simulink model "test"  (R2024b)
settings: Solver=VariableStepAuto  StartTime=0.0  StopTime=10.0  RelTol=1e-3
libraries: spsSeriesRLCLoadLib x6, spsAsynchronousMachineSIUnitsLib x4, spsUniversalBridgeLib x3, spsCurrentMeasurementLib x1, spsThreePhaseVIMeasurementLib x1, spsVoltageMeasurementLib x1
settings Model: Creator=HFUT2  LastModifiedBy=HFUT2

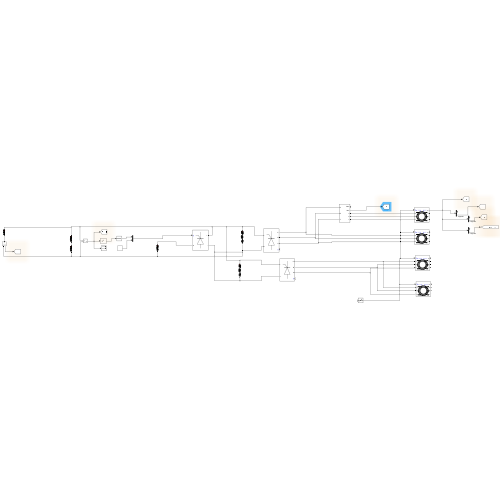
[thumbnail: Simulink's stored preview of the top-level diagram]
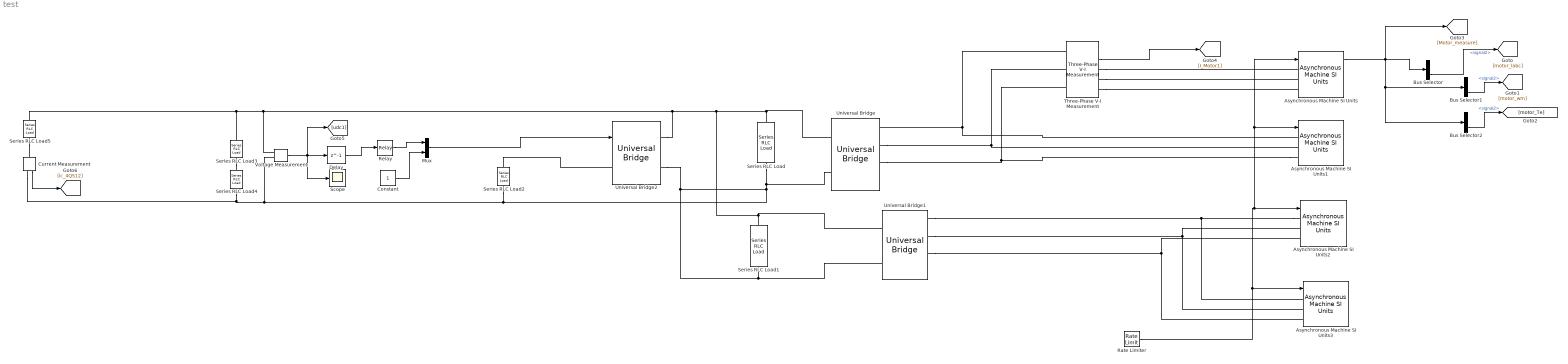
== system test ==
  Asynchronous Machine SI Units{,1..3} (4 alike) : spsAsynchronousMachineSIUnitsLib/Asynchronous Machine SI Units  RotorType=Wound  PresetModel=No  MechanicalLoad=Torque Tm  ShowDetailedParameters=on  ReferenceFrame=Rotor  Units=SI  MeasurementBus=off  NominalParameters=[1.845e+04 400 50]  VoltageRatio=1  Stator=[0.5968 0.0003495]  Rotor=[0.6258 0.005473]  Cage1=[0.4155 0.002066]  Cage2=[0.4168 0.0003495]  Lm=0.0354  Mechanical=[0.05 0.005879 2]  PolePairs=2  InitialConditions=[0 0 0 0 0 0 0 0]  SimulateSaturation=off  Saturation=[14.03593122, 27.81365428, 53.79336849, 72.68890987, 97.98006896, 148.6815601, 215.7428561, 302.9841135, 428.7778367 ; 230, 322, 414, 460, 506, 552, 598, 644, 690]  LoadFlowParameters=1492000  TsPowergui=0  TsBlock=-1  IterativeModel=Trapezoidal non iterative  IterativeDiscreteModel=Trapezoidal non iterative  Pmec=1.492e+006
  Bus Selector : BusSelector  OutputSignals=signal1,signal2
  Bus Selector1 : BusSelector  OutputSignals=signal1,signal2
  Bus Selector2 : BusSelector  OutputSignals=signal1,signal2
  Constant : Constant
  Current Measurement : spsCurrentMeasurementLib/Current Measurement  PhasorSimulation=off  OutputType=Complex  PSBequivalent=0
  Delay : Delay  DelayLength=1  InitialCondition=0
  Mux : Mux  Inputs=2
  Rate Limiter : RateLimiter  SampleTimeMode=inherited
  Relay : Relay
  Scope : Scope
  Series RLC Load{,1..5} (6 alike) : spsSeriesRLCLoadLib/Series RLC Load  LConnTagsString=a  RConnTagsString=__new0  NominalVoltage=1000  NominalFrequency=60  ActivePower=10e3  InductivePower=100  CapacitivePower=100  Setx0=off  InitialVoltage=0  SetiL0=off  InitialCurrent=0  Measurements=None  LoadType=constant Z
  Three-Phase V-I Measurement : spsThreePhaseVIMeasurementLib/Three-Phase V-I Measurement  VoltageMeasurement=phase-to-ground  SetLabelV=off  LabelV=Vabc  Vpu=off  VpuLL=off  CurrentMeasurement=yes  SetLabelI=off  LabelI=Iabc  Ipu=off  Pbase=100e6  Vbase=500e3  OutputType=Complex  PhasorSimulation=off  PSBequivalent=0
  Universal Bridge : spsUniversalBridgeLib/Universal Bridge  Arms=3  SnubberResistance=1e5  SnubberCapacitance=inf  Device=Thyristors  Ron=1e-3  Lon=0  ForwardVoltages="[  0  0  ]"  ForwardVoltage=0  GTOparameters=[ 10e-6 , 20e-6 ]  IGBTparameters=[ 1e-6 , 2e-6 ]  Measurements=None  Measurements_2=None  converterType=Rectifier
  Universal Bridge1 : spsUniversalBridgeLib/Universal Bridge  Arms=3  SnubberResistance=1e5  SnubberCapacitance=inf  Device=Thyristors  Ron=1e-3  Lon=0  ForwardVoltages="[  0  0  ]"  ForwardVoltage=0  GTOparameters=[ 10e-6 , 20e-6 ]  IGBTparameters=[ 1e-6 , 2e-6 ]  Measurements=None  Measurements_2=None  converterType=Rectifier
  Universal Bridge2 : spsUniversalBridgeLib/Universal Bridge  Arms=1  SnubberResistance=1e5  SnubberCapacitance=inf  Device=Thyristors  Ron=1e-3  Lon=0  ForwardVoltages="[  0  0  ]"  ForwardVoltage=0  GTOparameters=[ 10e-6 , 20e-6 ]  IGBTparameters=[ 1e-6 , 2e-6 ]  Measurements=None  Measurements_2=None  converterType=Rectifier
  Voltage Measurement : spsVoltageMeasurementLib/Voltage Measurement  PhasorSimulation=off  OutputType=Complex  PSBequivalent=0
  wires:
  Voltage Measurement/1 -> Scope/1, Delay/1, [udc1]
  Asynchronous Machine SI Units/1 -> Bus Selector2/1, Bus Selector1/1, Bus Selector/1, [Motor_measure]
  Three-Phase V-I Measurement/2 -> [I_Motor1]
  Rate Limiter/1 -> Asynchronous Machine SI Units1/1, Asynchronous Machine SI Units/1, Asynchronous Machine SI Units2/1, Asynchronous Machine SI Units3/1
  Mux/1 -> Universal Bridge2/1
  Relay/1 -> Mux/1
  Delay/1 -> Relay/1
  Bus Selector1/2 -> [motor_wm]  "<signal2>"
  Bus Selector2/2 -> [motor_Te]  "<signal2>"
  Current Measurement/1 -> [ic_4QS12]
  Bus Selector/2 -> [motor_labc]  "<signal2>"
  Constant/1 -> Mux/2
  connections:
  Universal Bridge2/RConn2 -- Universal Bridge1/RConn1 -- Series RLC Load1/RConn1 -- Series RLC Load/RConn1 -- Universal Bridge/RConn1 -- Current Measurement/RConn1 -- Series RLC Load4/RConn1 -- Voltage Measurement/LConn2 -- Series RLC Load2/RConn1
  Universal Bridge/RConn2 -- Series RLC Load/LConn1 -- Universal Bridge1/RConn2 -- Series RLC Load1/LConn1 -- Series RLC Load5/LConn1 -- Series RLC Load3/LConn1 -- Voltage Measurement/LConn1 -- Universal Bridge2/RConn1
  Asynchronous Machine SI Units3/LConn2 -- Universal Bridge1/LConn2 -- Asynchronous Machine SI Units2/LConn2
  Asynchronous Machine SI Units3/LConn3 -- Universal Bridge1/LConn1 -- Asynchronous Machine SI Units2/LConn3
  Universal Bridge/LConn3 -- Asynchronous Machine SI Units1/LConn1 -- Three-Phase V-I Measurement/LConn1
  Universal Bridge/LConn2 -- Three-Phase V-I Measurement/LConn2 -- Asynchronous Machine SI Units1/LConn2
  Asynchronous Machine SI Units2/LConn1 -- Universal Bridge1/LConn3 -- Asynchronous Machine SI Units3/LConn1
  Asynchronous Machine SI Units1/LConn3 -- Universal Bridge/LConn1 -- Three-Phase V-I Measurement/LConn3
  Universal Bridge2/LConn1 -- Series RLC Load2/LConn1
  Three-Phase V-I Measurement/RConn3 -- Asynchronous Machine SI Units/LConn3
  Three-Phase V-I Measurement/RConn1 -- Asynchronous Machine SI Units/LConn1
  Series RLC Load3/RConn1 -- Series RLC Load4/LConn1
  Series RLC Load5/RConn1 -- Current Measurement/LConn1
  Three-Phase V-I Measurement/RConn2 -- Asynchronous Machine SI Units/LConn2
